simulink library "fpga_utils_lib"  (R2023b)
settings: Solver=VariableStepAuto  StartTime=0.0  StopTime=10.0  RelTol=1e-3
undefined symbols (not defined in the file): a, b, Bias1, Bias2, c, DiscIntNeverNeededParam, NumBits1, NumBits2, Slope1, Slope2
libraries: simulink x8, hdlsllib x7, $bdroot x4
settings Model: Creator=promero  LastModifiedBy=promero
settings ModelReferenceCC: EnableRefExpFcnMdlSchedulingChecks=on

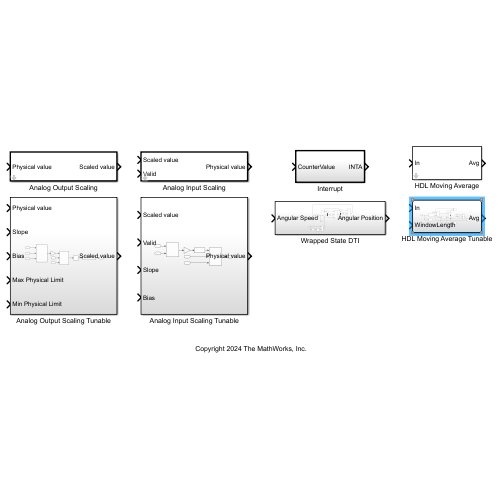
[thumbnail: Simulink's stored preview of the top-level diagram]
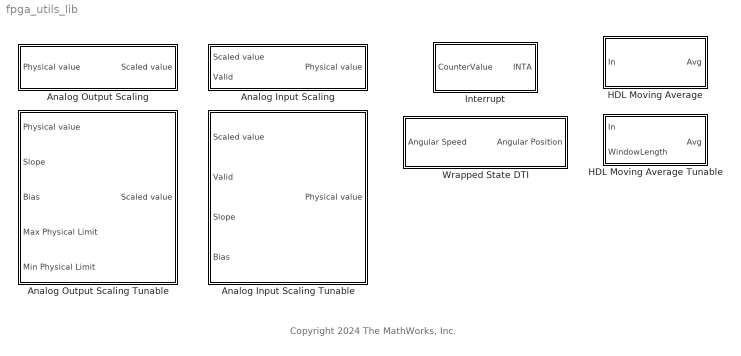
== system fpga_utils_lib ==
  note: Copyright 2024 The MathWorks, Inc.
  Analog Input Scaling : Subsystem  TreatAsAtomicUnit=on  mask(Analog Output Scaling){slope=1, bias=0}
      mask help: This block computes the analog linear scaling for a physical signal with support for slope and bias.
  Analog Input Scaling Tunable : Subsystem
  Analog Output Scaling : Subsystem  TreatAsAtomicUnit=on  mask(Analog Output Scaling){slope=1, bias=0, saturatePhys=off, maxPhysLim=inf, minPhysLim=-inf}
      mask prompts: saturatePhys "Saturate physical signal values"; maxPhysLim "Maximum physical limit"; minPhysLim "Minimum physical limit"
      mask help: This block computes the analog linear scaling for a physical signal with support for slope and bias.
      mask Callback saturatePhys:
      | % Control parameter visiblity
      | sat = get_param(gcb,'saturatePhys');
      | 
      | handle = get_param(gcb,'MaskObject');
      | contObj = handle.getDialogControl('ContainerLims');
      | 
      | % Set the 'MaskVisibilities' property for each parameters
      | if strcmp(sat,'on')
      |     contObj.Visible = 'on';
      | else
      |     contObj.Visible = 'off';
      |     set_param(gcb,'maxPhysLim','inf');
      |     set_param(gcb,'minPhysLim','-inf');
      | end
      mask DialogControl ContainerLims Prompt: Physical numerical limits
  Analog Output Scaling Tunable : Subsystem
  HDL Moving Average : Subsystem  mask{avgRatio=10}
      mask prompts: avgRatio "Window length"
  HDL Moving Average Tunable : Subsystem
  Interrupt : Subsystem  TreatAsAtomicUnit=on
  Wrapped State DTI : Subsystem

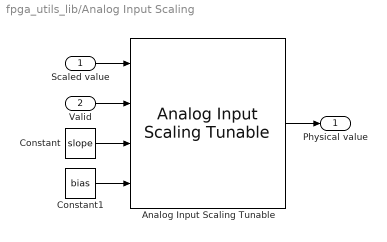
== system fpga_utils_lib/Analog Input Scaling ==
  Scaled value : Inport
  Valid : Inport  Port=2
  Analog Input Scaling Tunable : $bdroot/Analog Input Scaling Tunable  SystemSampleTime=-1  VariantActivationTime=update diagram  AllowFlexibleInterface=on  Latency=0  AutoFrameSizeCalculation=off
  Constant : Constant  Value=slope  SampleTime=-1
  Constant1 : Constant  Value=bias  SampleTime=-1
  Physical value : Outport
  wires:
  Analog Input Scaling Tunable/1 -> Physical value/1
  Constant1/1 -> Analog Input Scaling Tunable/4
  Constant/1 -> Analog Input Scaling Tunable/3
  Scaled value/1 -> Analog Input Scaling Tunable/1
  Valid/1 -> Analog Input Scaling Tunable/2

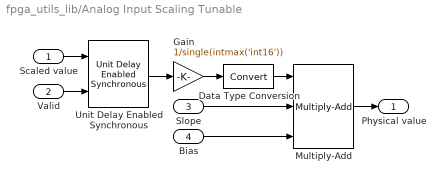
== system fpga_utils_lib/Analog Input Scaling Tunable ==
  Scaled value : Inport
  Valid : Inport  Port=2
  Slope : Inport  Port=3
  Bias : Inport  Port=4
  Data Type Conversion : DataTypeConversion  SaturateOnIntegerOverflow=off  RndMeth=Floor
  Gain : Gain  Gain=1/single(intmax('int16'))
  Multiply-Add : hdlsllib/HDL Operations/Multiply-Add  Function=c+(a.*b)  datatype=Inherit: Inherit via back propagation  DoSatur=off  FMA=off
  Unit Delay Enabled Synchronous : hdlsllib/Discrete/Unit Delay Enabled Synchronous  InitialCondition=0.0  SampleTime=-1
  Physical value : Outport
  wires:
  Bias/1 -> Multiply-Add/3
  Slope/1 -> Multiply-Add/2
  Gain/1 -> Data Type Conversion/1
  Multiply-Add/1 -> Physical value/1
  Unit Delay Enabled Synchronous/1 -> Gain/1
  Scaled value/1 -> Unit Delay Enabled Synchronous/1
  Valid/1 -> Unit Delay Enabled Synchronous/2
  Data Type Conversion/1 -> Multiply-Add/1

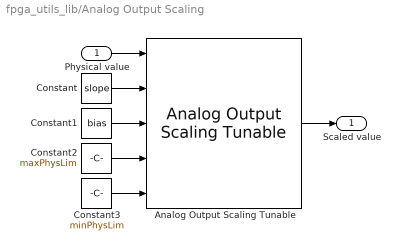
== system fpga_utils_lib/Analog Output Scaling ==
  Physical value : Inport
  Analog Output Scaling Tunable : $bdroot/Analog Output Scaling Tunable  SystemSampleTime=-1  VariantActivationTime=update diagram  AllowFlexibleInterface=on  Latency=0  AutoFrameSizeCalculation=off
  Constant : Constant  Value=slope  OutDataTypeStr=Inherit: Inherit via back propagation  SampleTime=-1
  Constant1 : Constant  Value=bias  OutDataTypeStr=Inherit: Inherit via back propagation  SampleTime=-1
  Constant2 : Constant  Value=maxPhysLim  OutDataTypeStr=Inherit: Inherit via back propagation  SampleTime=-1
  Constant3 : Constant  Value=minPhysLim  OutDataTypeStr=Inherit: Inherit via back propagation  SampleTime=-1
  Scaled value : Outport
  wires:
  Constant3/1 -> Analog Output Scaling Tunable/5
  Constant2/1 -> Analog Output Scaling Tunable/4
  Constant1/1 -> Analog Output Scaling Tunable/3
  Constant/1 -> Analog Output Scaling Tunable/2
  Analog Output Scaling Tunable/1 -> Scaled value/1
  Physical value/1 -> Analog Output Scaling Tunable/1

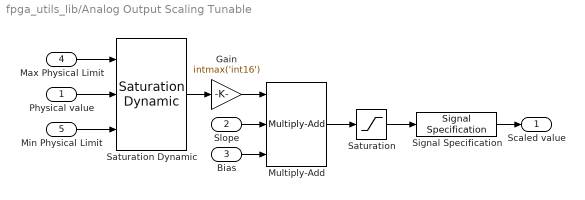
== system fpga_utils_lib/Analog Output Scaling Tunable ==
  Physical value : Inport
  Slope : Inport  Port=2
  Bias : Inport  Port=3
  Max Physical Limit : Inport  Port=4
  Min Physical Limit : Inport  Port=5
  Gain : Gain  Gain=intmax('int16')
  Multiply-Add : hdlsllib/HDL Operations/Multiply-Add  Function=c+(a.*b)  datatype=Inherit: Inherit via back propagation  DoSatur=off  FMA=off
  Saturation : Saturate  UpperLimit=intmax('int16')  LowerLimit=intmin('int16')
  Saturation Dynamic : simulink/Discontinuities/Saturation Dynamic  OutMin=[]  OutMax=[]  OutDataTypeStr=Inherit: Inherit via back propagation  OutDataType=fixdt(1, 16)  OutScaling=2^-10  DoSatur=off
  Signal Specification : SignalSpecification  OutDataTypeStr=int16
  Scaled value : Outport
  wires:
  Min Physical Limit/1 -> Saturation Dynamic/3
  Max Physical Limit/1 -> Saturation Dynamic/1
  Physical value/1 -> Saturation Dynamic/2
  Saturation Dynamic/1 -> Gain/1
  Saturation/1 -> Signal Specification/1
  Signal Specification/1 -> Scaled value/1
  Gain/1 -> Multiply-Add/1
  Slope/1 -> Multiply-Add/2
  Multiply-Add/1 -> Saturation/1
  Bias/1 -> Multiply-Add/3

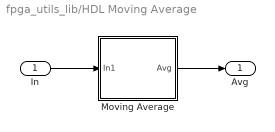
== system fpga_utils_lib/HDL Moving Average ==
  In : Inport
  Moving Average : Subsystem  Variant=on  VariantControl=Moving Average
  Avg : Outport
  wires:
  In/1 -> Moving Average/1(In1)
  Moving Average/1(Avg) -> Avg/1

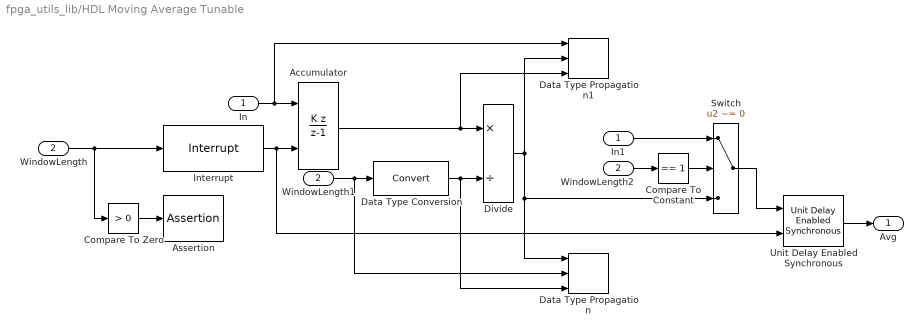
== system fpga_utils_lib/HDL Moving Average Tunable ==
  In : Inport
  WindowLength : Inport  Port=2
  Accumulator : DiscreteIntegrator  IntegratorMethod=Accumulation: Backward Euler  ExternalReset=falling  SampleTime=-1  OutDataTypeStr=Inherit: Inherit via back propagation  ICPrevOutput=DiscIntNeverNeededParam  ICPrevScaledInput=DiscIntNeverNeededParam
  Assertion : Assertion
  Compare To Constant : simulink/Logic and Bit Operations/Compare To Constant  relop===  const=1  OutDataTypeStr=boolean
  Compare To Zero : simulink/Logic and Bit Operations/Compare To Zero  relop=>  OutDataTypeStr=boolean
  Data Type Propagation : simulink/Signal Attributes/Data Type Propagation  PropDataType=fixdt(1, 16)  IfRefDouble=double  IfRefSingle=single  IsSigned=IsSigned2  NumBitsBase=NumBits2  NumBitsMult=1  NumBitsAdd=0  NumBitsAllowFinal=1:128  PropScaling=2^-10  ValuesUsedBestPrec=[5 -7]  SlopeBase=Slope2  SlopeMult=1  SlopeAdd=0  BiasBase=Bias2  BiasMult=1  BiasAdd=0
  Data Type Propagation1 : simulink/Signal Attributes/Data Type Propagation  PropDataType=fixdt(1, 16)  IfRefDouble=double  IfRefSingle=single  IsSigned=IsSigned1 or IsSigned2  NumBitsBase=NumBits1+NumBits2  NumBitsMult=1  NumBitsAdd=0  NumBitsAllowFinal=1:128  PropScaling=2^-10  ValuesUsedBestPrec=[5 -7]  SlopeBase=max([Slope1 Slope2])  SlopeMult=1  SlopeAdd=0  BiasBase=max([Bias1 Bias2])  BiasMult=1  BiasAdd=0
  Data Type Conversion : DataTypeConversion  SaturateOnIntegerOverflow=off  RndMeth=Floor
  Divide : Product  Inputs=*/  OutDataTypeStr=Inherit: Inherit via back propagation  RndMeth=Simplest  SaturateOnIntegerOverflow=on
  In1 : InportShadow
  Interrupt : $bdroot/Interrupt  SystemSampleTime=-1  VariantActivationTime=update diagram  AllowFlexibleInterface=on  Latency=0  AutoFrameSizeCalculation=off
  Switch : Switch  Criteria=u2 ~= 0  SaturateOnIntegerOverflow=off
  Unit Delay Enabled Synchronous : hdlsllib/Discrete/Unit Delay Enabled Synchronous  InitialCondition=0.0  SampleTime=-1
  WindowLength1 : InportShadow  Port=2
  WindowLength2 : InportShadow  Port=2
  Avg : Outport
  wires:
  In1/1 -> Switch/1
  WindowLength2/1 -> Compare To Constant/1
  Compare To Constant/1 -> Switch/2
  Switch/1 -> Unit Delay Enabled Synchronous/1
  Compare To Zero/1 -> Assertion/1
  Data Type Conversion/1 -> Data Type Propagation/3, Divide/2
  Divide/1 -> Data Type Propagation1/2, Data Type Propagation/1, Switch/3
  Unit Delay Enabled Synchronous/1 -> Avg/1
  In/1 -> Data Type Propagation1/1, Accumulator/1
  Interrupt/1 -> Unit Delay Enabled Synchronous/2, Accumulator/2
  WindowLength1/1 -> Data Type Propagation/2, Data Type Conversion/1
  WindowLength/1 -> Compare To Zero/1, Interrupt/1
  Accumulator/1 -> Data Type Propagation1/3, Divide/1

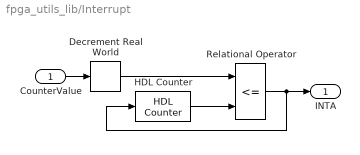
== system fpga_utils_lib/Interrupt ==
  CounterValue : Inport
  Decrement Real World : hdlsllib/Math Operations/Decrement Real World
  HDL Counter : hdlsllib/Sources/HDL Counter  CountType=Free running  CountInit=0  CountStep=1  CountMax=25  CountFromType=Initial value  CountFrom=0  CountResetPort=on  CountLoadPort=off  CountEnbPort=off  CountDirPort=off  CountHitOutputPort=off  CountDataType=Unsigned  CountWordLen=32  CountFracLen=0  CountSampTime=1
  Relational Operator : RelationalOperator  Operator=<=  OutDataTypeStr=boolean  RndMeth=Simplest  InputSameDT=off
  INTA : Outport  VectorParamsAs1DForOutWhenUnconnected=off
  wires:
  Relational Operator/1 -> HDL Counter/1, INTA/1
  Decrement Real World/1 -> Relational Operator/1
  HDL Counter/1 -> Relational Operator/2
  CounterValue/1 -> Decrement Real World/1

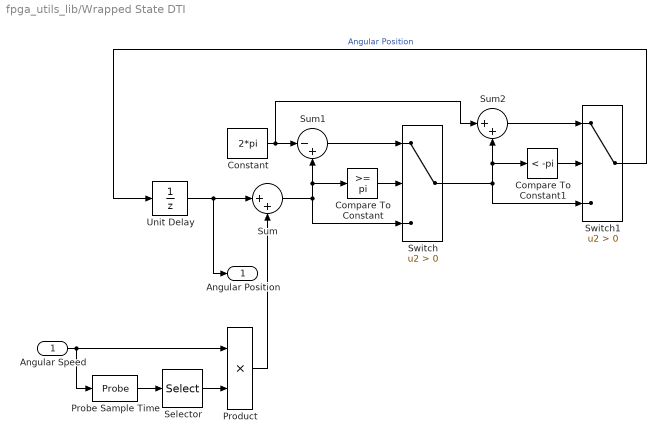
== system fpga_utils_lib/Wrapped State DTI ==
  Angular Speed : Inport
  Compare To Constant : simulink/Logic and Bit Operations/Compare To Constant  relop=>=  const=pi  OutDataTypeStr=boolean
  Compare To Constant1 : simulink/Logic and Bit Operations/Compare To Constant  relop=<  const=-pi  OutDataTypeStr=boolean
  Constant : Constant  Value=2*pi  OutDataTypeStr=Inherit: Inherit via back propagation  SampleTime=-1
  Probe Sample Time : Probe  ProbeWidth=off  ProbeComplexSignal=off  ProbeSampleTimeDataType=Same as input
  Product : Product
  Selector : Selector  InputPortWidth=2  IndexOptions=Index vector (dialog)  Indices=1  OutputSizes=1
  Sum : Sum  Inputs=|++
  Sum1 : Sum  Inputs=|-+
  Sum2 : Sum  Inputs=|++
  Switch : Switch  Criteria=u2 > Threshold  SaturateOnIntegerOverflow=off  InputSameDT=off
  Switch1 : Switch  Criteria=u2 > Threshold  SaturateOnIntegerOverflow=off  InputSameDT=off
  Unit Delay : UnitDelay  SampleTime=-1  HasFrameUpgradeWarning=on
  Angular Position : Outport
  wires:
  Compare To Constant1/1 -> Switch1/2
  Unit Delay/1 -> Sum/1, Angular Position/1
  Constant/1 -> Sum2/1, Sum1/1
  Sum2/1 -> Switch1/1
  Switch1/1 -> Unit Delay/1  "Angular Position"
  Switch/1 -> Sum2/2, Compare To Constant1/1, Switch1/3
  Compare To Constant/1 -> Switch/2
  Sum/1 -> Compare To Constant/1, Sum1/2, Switch/3
  Sum1/1 -> Switch/1
  Angular Speed/1 -> Probe Sample Time/1, Product/1
  Probe Sample Time/1 -> Selector/1
  Product/1 -> Sum/2
  Selector/1 -> Product/2

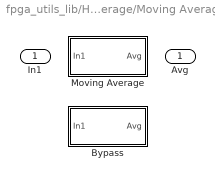
== system fpga_utils_lib/HDL Moving Average/Moving Average ==
  In1 : Inport
  Bypass : Subsystem  VariantControl=avgRatio == 1
  Moving Average : Subsystem  VariantControl=avgRatio > 1
  Avg : Outport

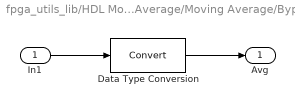
== system fpga_utils_lib/HDL Moving Average/Moving Average/Bypass ==
  In1 : Inport
  Data Type Conversion : DataTypeConversion  SaturateOnIntegerOverflow=off  RndMeth=Floor
  Avg : Outport
  wires:
  In1/1 -> Data Type Conversion/1
  Data Type Conversion/1 -> Avg/1

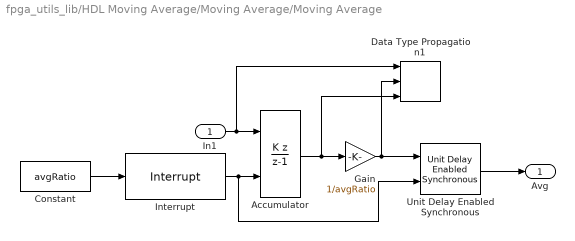
== system fpga_utils_lib/HDL Moving Average/Moving Average/Moving Average ==
  In1 : Inport
  Accumulator : DiscreteIntegrator  IntegratorMethod=Accumulation: Backward Euler  ExternalReset=falling  SampleTime=-1  OutDataTypeStr=Inherit: Inherit via back propagation  ICPrevOutput=DiscIntNeverNeededParam  ICPrevScaledInput=DiscIntNeverNeededParam
  Constant : Constant  Value=avgRatio  OutDataTypeStr=uint16  SampleTime=-1  LockScale=on
  Data Type Propagation1 : simulink/Signal Attributes/Data Type Propagation  PropDataType=fixdt(1, 16)  IfRefDouble=double  IfRefSingle=single  IsSigned=IsSigned1 or IsSigned2  NumBitsBase=NumBits1+NumBits2  NumBitsMult=1  NumBitsAdd=0  NumBitsAllowFinal=1:128  PropScaling=2^-10  ValuesUsedBestPrec=[5 -7]  SlopeBase=max([Slope1 Slope2])  SlopeMult=1  SlopeAdd=0  BiasBase=max([Bias1 Bias2])  BiasMult=1  BiasAdd=0
  Gain : Gain  Gain=1/avgRatio  OutDataTypeStr=Inherit: Inherit via back propagation  LockScale=on
  Interrupt : $bdroot/Interrupt  SystemSampleTime=-1  VariantActivationTime=update diagram  AllowFlexibleInterface=on  Latency=0  AutoFrameSizeCalculation=off
  Unit Delay Enabled Synchronous : hdlsllib/Discrete/Unit Delay Enabled Synchronous  InitialCondition=0.0  SampleTime=-1
  Avg : Outport
  wires:
  Interrupt/1 -> Unit Delay Enabled Synchronous/2, Accumulator/2
  Accumulator/1 -> Data Type Propagation1/3, Gain/1
  In1/1 -> Data Type Propagation1/1, Accumulator/1
  Gain/1 -> Data Type Propagation1/2, Unit Delay Enabled Synchronous/1
  Unit Delay Enabled Synchronous/1 -> Avg/1
  Constant/1 -> Interrupt/1
